simulink model "Maglev_model_discreto"  (R2023b)
settings: Solver=VariableStepAuto  StartTime=0.0  StopTime=3.0  RelTol=1e-3
values from neighbouring files (symbols this model uses):
  d1 = C_d_simple.Denominator{1,1}(2)    [ControladoresSimulink.m]
  d2 = d1d2/d1    [ControladoresSimulink.m]
  gamma = 328    [planta_maglev.m]
  ki = 2*g / i0    (= 20.6809318014)    [planta_maglev.m]
  kx = -2*g / x0    (= -860.526315789)    [planta_maglev.m]
  p = C_d_simple.Numerator{1,1}(1)    [ControladoresSimulink.m]
  q = qd1/d1    [ControladoresSimulink.m]
  r = rd1d2/d1    [ControladoresSimulink.m]
  rho = 0.166    [planta_maglev.m]
  Ts = 2e-4    (= 0.0002)    [ControladoresSimulink.m]
libraries: slpidlib x1, cstblocks x1
settings Model: PacingRate=10  Creator=chris  LastModifiedBy=chris

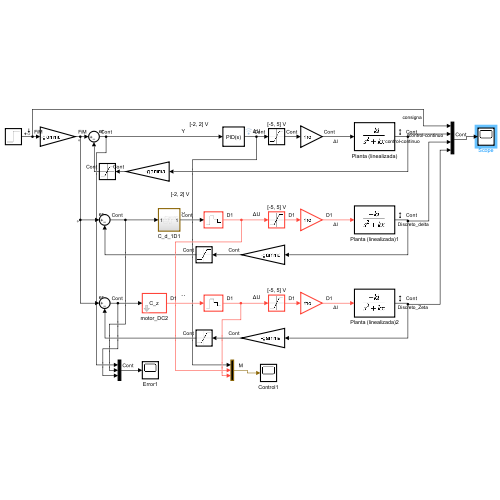
[thumbnail: Simulink's stored preview of the top-level diagram]
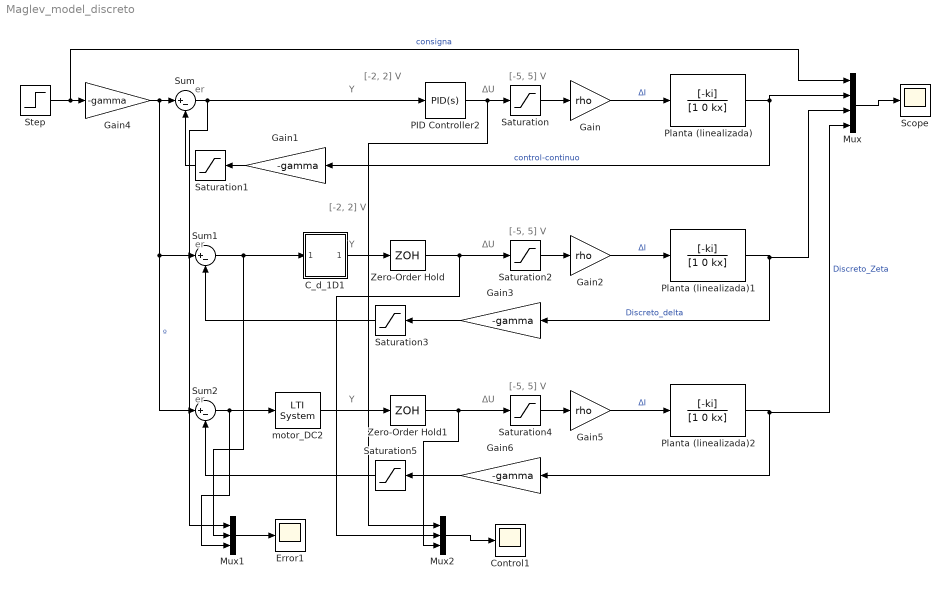
== system Maglev_model_discreto ==
  note: [-2, 2] V
  note: [-5, 5] V
  note: Y
  note: ΔU
  note: er
  note: Y
  note: [-2, 2] V
  note: ΔU
  note: er
  note: [-5, 5] V
  note: Y
  note: ΔU
  note: [-5, 5] V
  note: er
  C_d_1D1 : Subsystem
  Control1 : Scope
  Error1 : Scope
  Gain : Gain  Gain=rho
  Gain{1,3..4,6} (4 alike) : Gain  Gain=-gamma
  Gain2 : Gain  Gain=rho
  Gain5 : Gain  Gain=rho
  Mux : Mux
  Mux1 : Mux  Inputs=3
  Mux2 : Mux  Inputs=3
  PID Controller2 : slpidlib/PID Controller  Controller=PID  Form=Parallel  TimeDomain=Continuous-time  UseExternalTs=off  SampleTime=-1  IntegratorMethod=Forward Euler  FilterMethod=Forward Euler  ControllerParametersSource=internal  P=18.4157926253428  I=66.574639801784  UseKiTs=off  D=0.401108645856644  N=51667.197865857  UseFilter=on  TunerSelectOption=Transfer Function Based (PID Tuner App)  InitialConditionSource=internal  InitialConditionForIntegrator=0  InitialConditionForFilter=0  DifferentiatorICPrevScaledInput=0  ExternalReset=none  TrackingMode=off  Kt=1  LimitOutput=off  SatLimitsSource=internal  UpperSaturationLimit=5  LowerSaturationLimit=-5  LinearizeAsGain=on  AntiWindupMode=back-calculation  Kb=1  LimitIntegrator=off  UpperIntegratorSaturationLimit=inf  LowerIntegratorSaturationLimit=-inf  POutMin=[]  POutMax=[]  IOutMin=[]  IOutMax=[]  DOutMin=[]  DOutMax=[]  NOutMin=[]  NOutMax=[]  SumOutMin=[]  SumOutMax=[]  SaturationOutMin=[]  SaturationOutMax=[]  PParamMin=[]  PParamMax=[]  IParamMin=[]  IParamMax=[]  DParamMin=[]  DParamMax=[]  NParamMin=[]  NParamMax=[]  KbParamMin=[]  KbParamMax=[]  KtParamMin=[]  KtParamMax=[]  KbOutMin=[]  KbOutMax=[]  KtOutMin=[]  KtOutMax=[]  IntegratorOutMin=[]  IntegratorOutMax=[]  FilterOutMin=[]  FilterOutMax=[]  SumI1OutMin=[]  SumI1OutMax=[]  SumI2OutMin=[]  SumI2OutMax=[]  SumI3OutMin=[]  SumI3OutMax=[]  SumI4OutMin=[]  SumI4OutMax=[]  SumDOutMin=[]  SumDOutMax=[]  DifferentiatorOutMin=[]  DifferentiatorOutMax=[]  FilterDiffOutCoefMin=[]  FilterDiffOutCoefMax=[]  ReciprocalOutMin=[]  ReciprocalOutMax=[]  SumDenOutMin=[]  SumDenOutMax=[]  SumNumOutMin=[]  SumNumOutMax=[]  DivideOutMin=[]  DivideOutMax=[]  UdiffTsProdOutMin=[]  UdiffTsProdOutMax=[]  NTsProdOutMin=[]  NTsProdOutMax=[]  UintegralTsProdOutMin=[]  UintegralTsProdOutMax=[]  UngainTsProdOutMin=[]  UngainTsProdOutMax=[]  ClampingZeroOutDataTypeStr=Inherit: Inherit via back propagation  ClampingZeroOutMin=[]  ClampingZeroOutMax=[]  FilterDenConstantOutDataTypeStr=Inherit: Inherit via back propagation  FilterDenConstantOutMin=[]  FilterDenConstantOutMax=[]  PCopyOutDataTypeStr=Inherit: Inherit via back propagation  PCopyOutMin=[]  PCopyOutMax=[]  NCopyOutDataTypeStr=Inherit: Inherit via back propagation  NCopyOutMin=[]  NCopyOutMax=[]  IntegratorContinuousStateAttributes=''  IntegratorStateMustResolveToSignalObject=off  IntegratorRTWStateStorageClass=Auto  FilterContinuousStateAttributes=''  FilterStateMustResolveToSignalObject=off  FilterRTWStateStorageClass=Auto  ParallelPVariant=InternalParameters  IdealPVariant=Disabled  IVariant=InternalParameters  DVariant=InternalParameters  IntegratorVariant=Continuous  SatVariant=Disabled  AWVariant=Passthrough  PCopyVariant=Disabled  TRVariant=Disabled  FdbkBlocksVariant=Forward  IdealPFdbkVariant=Disabled  SatFdbkVariant=Disabled  DerivativeFilterVariant=ContFilter  NVariant=InternalParameters  NCopyVariant=Disabled  FilterICVariant=InternalICsFilter  IntegratorICVariant=InternalICs  ExternalResetVariant=Disabled  TRSumVariant=Passthrough  SumFdbkVariant=Disabled  SumVariant=Sum_PID  TsampFilterVariant=InternalTs  TsampNgainVariant=Passthrough  TsampIntegralVariant=Disabled_SignalSpec  ExternalSaturationOutDataTypeStr=Inherit: Same as second input
  Planta (linealizada) : TransferFcn  Numerator=[-ki]  Denominator=[1 0 kx]
  Planta (linealizada)1 : TransferFcn  Numerator=[-ki]  Denominator=[1 0 kx]
  Planta (linealizada)2 : TransferFcn  Numerator=[-ki]  Denominator=[1 0 kx]
  Saturation : Saturate  UpperLimit=5  LowerLimit=-5
  Saturation1 : Saturate  UpperLimit=2  LowerLimit=-2
  Saturation2 : Saturate  UpperLimit=5  LowerLimit=-5
  Saturation3 : Saturate  UpperLimit=2  LowerLimit=-2
  Saturation4 : Saturate  UpperLimit=5  LowerLimit=-5
  Saturation5 : Saturate  UpperLimit=2  LowerLimit=-2
  Scope : Scope
  Step : Step  Before=-0.005  After=0.004  SampleTime=0
  Sum : Sum  Inputs=|+-
  Sum1 : Sum  Inputs=|+-
  Sum2 : Sum  Inputs=|+-
  Zero-Order Hold : ZeroOrderHold  SampleTime=Ts
  Zero-Order Hold1 : ZeroOrderHold  SampleTime=Ts
  motor_DC2 : cstblocks/LTI System  sys=C_z  IC=[]  PadeOrder=0
  wires:
  PID Controller2/1 -> Mux2/1, Saturation/1
  Gain1/1 -> Saturation1/1
  Saturation1/1 -> Sum/2
  Saturation/1 -> Gain/1
  Gain/1 -> Planta (linealizada)/1  "ΔI"
  Sum/1 -> Mux1/1, PID Controller2/1
  Step/1 -> Mux/1, Gain4/1  "consigna"
  Planta (linealizada)/1 -> Mux/2, Gain1/1  "control-continuo"
  Mux/1 -> Scope/1
  Planta (linealizada)1/1 -> Mux/3, Gain3/1  "Discreto_delta"
  Gain2/1 -> Planta (linealizada)1/1  "ΔI"
  Gain3/1 -> Saturation3/1
  Saturation2/1 -> Gain2/1
  Sum1/1 -> Mux1/2, C_d_1D1/1(In1)
  Saturation3/1 -> Sum1/2
  C_d_1D1/1(Out1) -> Zero-Order Hold/1
  Zero-Order Hold/1 -> Mux2/2, Saturation2/1
  Zero-Order Hold1/1 -> Mux2/3, Saturation4/1
  Gain4/1 -> Sum2/1, Sum1/1, Sum/1  "º"
  Planta (linealizada)2/1 -> Mux/4, Gain6/1  "Discreto_Zeta"
  Saturation4/1 -> Gain5/1
  Gain5/1 -> Planta (linealizada)2/1  "ΔI"
  Gain6/1 -> Saturation5/1
  Saturation5/1 -> Sum2/2
  motor_DC2/1 -> Zero-Order Hold1/1
  Mux1/1 -> Error1/1
  Sum2/1 -> motor_DC2/1, Mux1/3
  Mux2/1 -> Control1/1

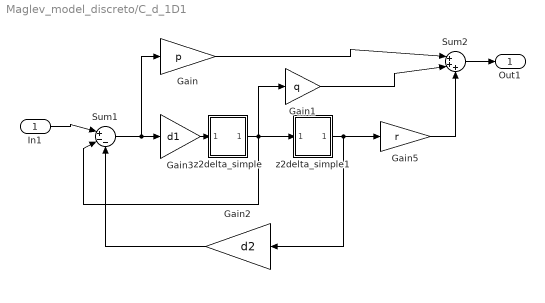
== system Maglev_model_discreto/C_d_1D1 ==
  In1 : Inport
  Gain : Gain  Gain=p
  Gain1 : Gain  Gain=q
  Gain2 : Gain  Gain=d2
  Gain3 : Gain  Gain=d1
  Gain5 : Gain  Gain=r
  Sum1 : Sum  Inputs=|+--
  Sum2 : Sum  Inputs=|+++
  z2delta_simple : Subsystem
  z2delta_simple1 : Subsystem
  Out1 : Outport
  wires:
  In1/1 -> Sum1/1
  Gain1/1 -> Sum2/2
  Gain5/1 -> Sum2/3
  Gain/1 -> Sum2/1
  Sum2/1 -> Out1/1
  z2delta_simple1/1(Out1) -> Gain2/1, Gain5/1
  Sum1/1 -> Gain/1, Gain3/1
  z2delta_simple/1(Out1) -> Gain1/1, Sum1/2, z2delta_simple1/1(In1)
  Gain2/1 -> Sum1/3
  Gain3/1 -> z2delta_simple/1(In1)

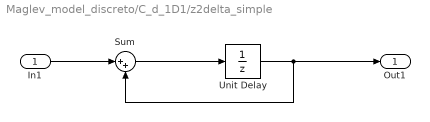
== system Maglev_model_discreto/C_d_1D1/z2delta_simple ==
  In1 : Inport
  Sum : Sum  Inputs=|++
  Unit Delay : UnitDelay  SampleTime=-1  HasFrameUpgradeWarning=on
  Out1 : Outport
  wires:
  In1/1 -> Sum/1
  Unit Delay/1 -> Out1/1, Sum/2
  Sum/1 -> Unit Delay/1

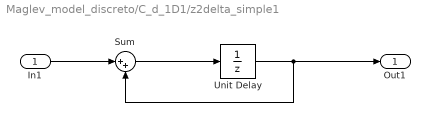
== system Maglev_model_discreto/C_d_1D1/z2delta_simple1 ==
  In1 : Inport
  Sum : Sum  Inputs=|++
  Unit Delay : UnitDelay  SampleTime=-1  HasFrameUpgradeWarning=on
  Out1 : Outport
  wires:
  In1/1 -> Sum/1
  Unit Delay/1 -> Out1/1, Sum/2
  Sum/1 -> Unit Delay/1
